simulink model "Vfinal"  (R2023b)
settings: Solver=VariableStepAuto  StartTime=0.0  StopTime=10.0  RelTol=1e-3
settings Model: Creator=meghn  LastModifiedBy=Hp

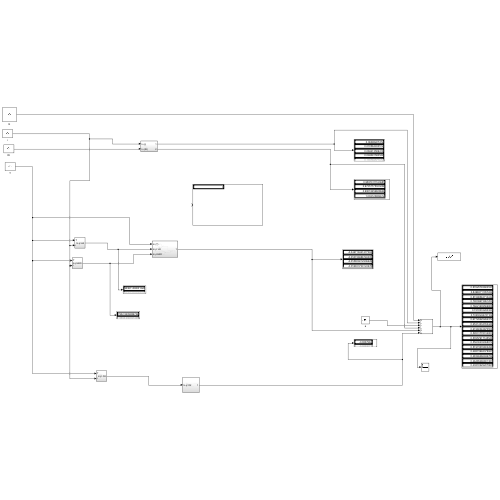
[thumbnail: Simulink's stored preview of the top-level diagram]
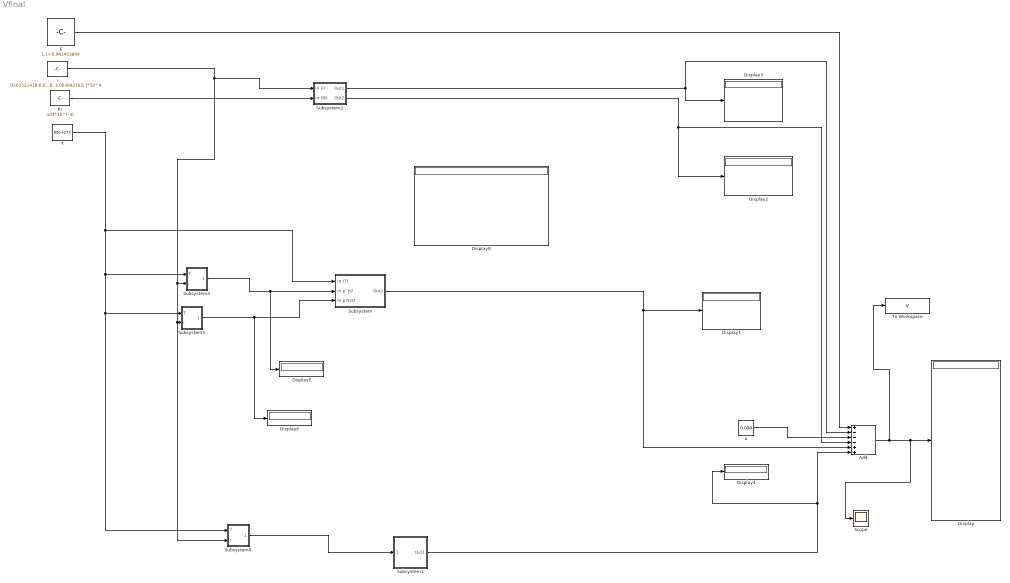
== system Vfinal ==
  Add : Sum  Inputs=+---++
  Display{,1..6,8} (8 alike) : Display
  E : Constant  Value=1.1+0.941453849
  Ri : Constant  Value=.104*10^(-4)
  Scope : Scope
  Subsystem : Subsystem
  Subsystem1 : Subsystem
  Subsystem2 : Subsystem
  Subsystem4 : Subsystem
  Subsystem5 : Subsystem
  Subsystem6 : Subsystem
  T : Constant  Value=800+273
  To Workspace : ToWorkspace  VariableName=V  SampleTime=-1
      settings: Save2DSignal=2-D array (concatenate along first dimension)
  a : Constant  Value=0.094
  i : Constant  Value=|
      | [0.61521418;0.697932053;
      | 0.811669129;
      | 0.904726736;
      | 0.997784343;
      | 1.158050222;
      | 1.26661743;
      | 1.380354505;
      | 1.499261448;
      | 1.659527326;
      | 1.783604136;
      | 1.88183161;
      | 1.990398818;
      | 2.192023634;
      | 2.310930576;
      | 2.398818316;
      | 2.507385524;
      | 2.662481536;
      | 3.003692762;
      | ]*10^4
  wires:
  a/1 -> Add/3
  T/1 -> Subsystem6/1(T), Subsystem5/1(T), Subsystem4/1(T), Subsystem/1(In (T))
  Subsystem4/1(In p' H2) -> Display5/1, Subsystem/2(In p' H2)
  Subsystem5/1(In p'H2O) -> Display6/1, Subsystem/3(In p'H2O)
  Subsystem/1(Out1) -> Display1/1, Add/5
  Subsystem1/1(Out1) -> Display4/1, Add/6
  Subsystem6/1(In p' O2) -> Subsystem1/1(In p' O2)
  Subsystem2/2(Out2) -> Display2/1, Add/4
  Subsystem2/1(Out1) -> Add/2, Display3/1
  i/1 -> Subsystem6/2(i), Subsystem5/2(i), Subsystem4/2(i), Subsystem2/1(In (i))
  Ri/1 -> Subsystem2/2(In (Ri))
  E/1 -> Add/1
  Add/1 -> To Workspace/1, Scope/1, Display/1

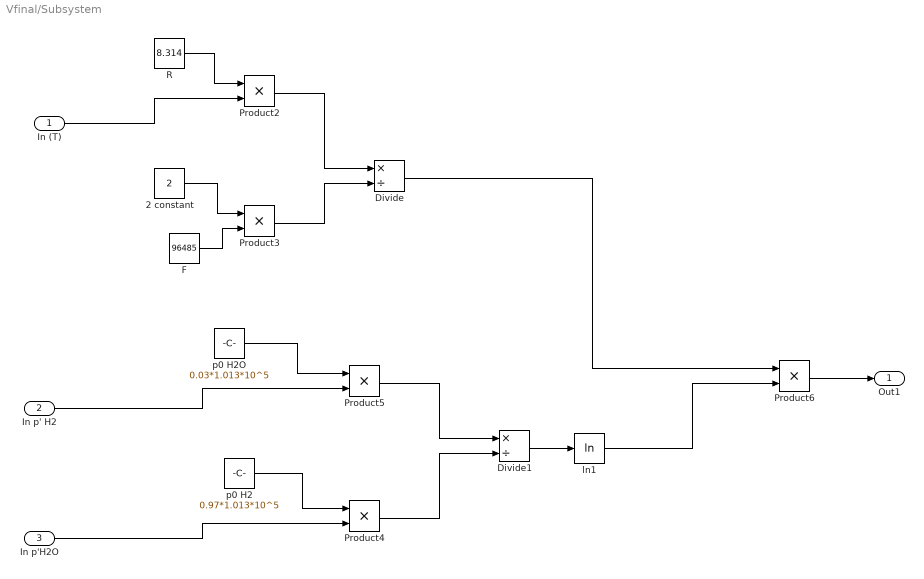
== system Vfinal/Subsystem ==
  In (T) : Inport
  In p' H2 : Inport  Port=2
  In p'H2O : Inport  Port=3
  2 constant : Constant  Value=2
  Divide : Product  Inputs=*/
  Divide1 : Product  Inputs=*/
  F : Constant  Value=96485
  Product{2..6} (5 alike) : Product
  R : Constant  Value=8.314
  ln1 : Math  Operator=log
  p0 H2 : Constant  Value=0.97*1.013*10^5
  p0 H2O : Constant  Value=0.03*1.013*10^5
  Out1 : Outport
  wires:
  Product5/1 -> Divide1/1
  Product4/1 -> Divide1/2
  R/1 -> Product2/1
  ln1/1 -> Product6/2
  In p' H2/1 -> Product5/2
  F/1 -> Product3/2
  Product3/1 -> Divide/2
  p0 H2/1 -> Product4/1
  Divide1/1 -> ln1/1
  p0 H2O/1 -> Product5/1
  Divide/1 -> Product6/1
  2 constant/1 -> Product3/1
  Product2/1 -> Divide/1
  In p'H2O/1 -> Product4/2
  In (T)/1 -> Product2/2
  Product6/1 -> Out1/1

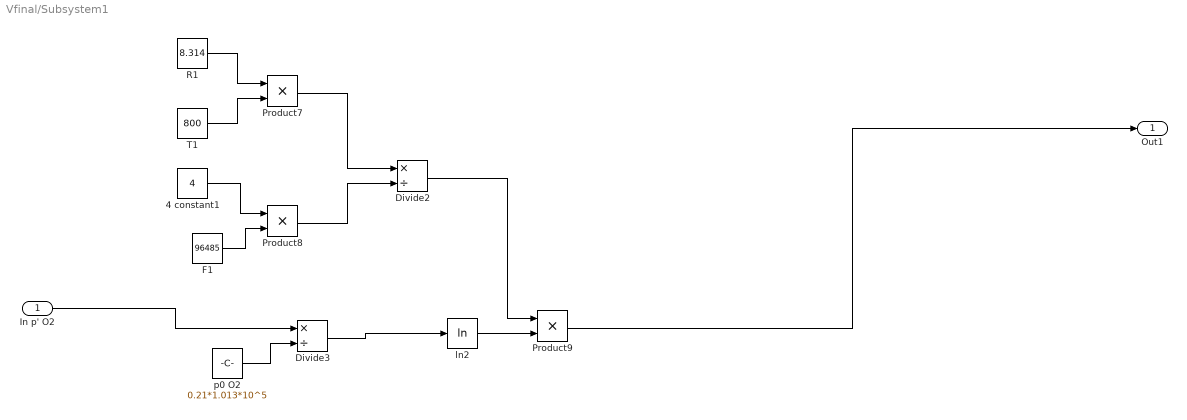
== system Vfinal/Subsystem1 ==
  In p' O2 : Inport
  4 constant1 : Constant  Value=4
  Divide2 : Product  Inputs=*/
  Divide3 : Product  Inputs=*/
  F1 : Constant  Value=96485
  Product7 : Product
  Product8 : Product
  Product9 : Product
  R1 : Constant  Value=8.314
  T1 : Constant  Value=800
  ln2 : Math  Operator=log
  p0 O2 : Constant  Value=0.21*1.013*10^5
  Out1 : Outport
  wires:
  ln2/1 -> Product9/2
  4 constant1/1 -> Product8/1
  R1/1 -> Product7/1
  Divide2/1 -> Product9/1
  p0 O2/1 -> Divide3/2
  F1/1 -> Product8/2
  T1/1 -> Product7/2
  Divide3/1 -> ln2/1
  Product8/1 -> Divide2/2
  Product7/1 -> Divide2/1
  In p' O2/1 -> Divide3/1
  Product9/1 -> Out1/1

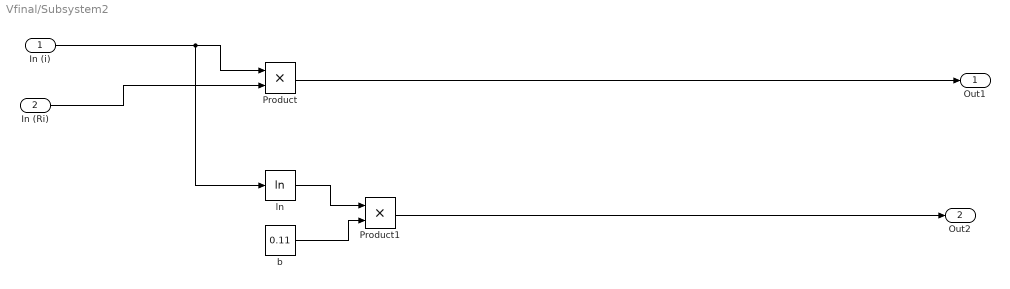
== system Vfinal/Subsystem2 ==
  In (i) : Inport
  In (Ri) : Inport  Port=2
  Product : Product
  Product1 : Product
  b : Constant  Value=0.11
  ln : Math  Operator=log
  Out1 : Outport
  Out2 : Outport  Port=2
  wires:
  b/1 -> Product1/2
  ln/1 -> Product1/1
  Product1/1 -> Out2/1
  In (Ri)/1 -> Product/2
  In (i)/1 -> ln/1, Product/1
  Product/1 -> Out1/1

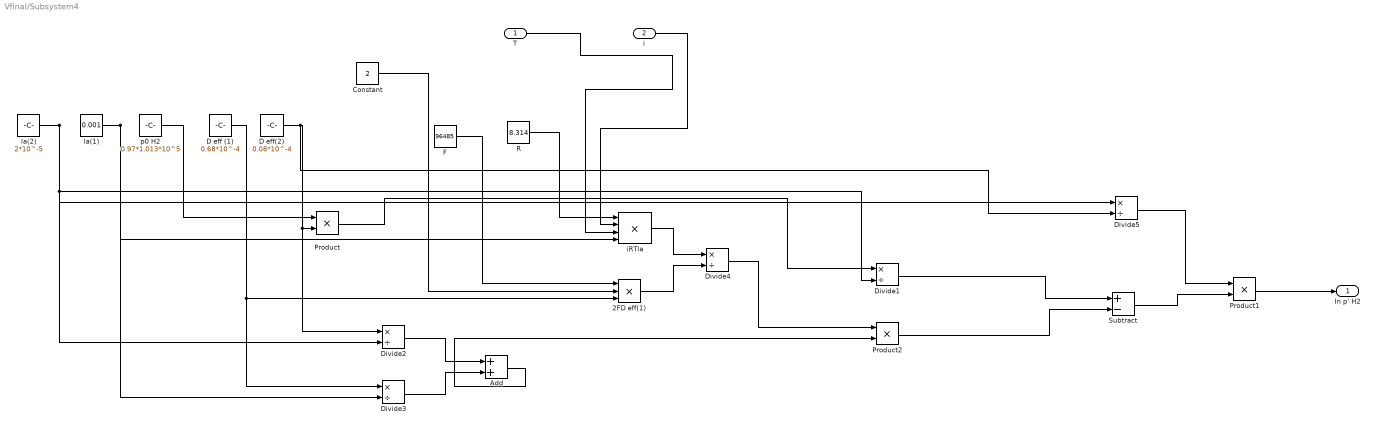
== system Vfinal/Subsystem4 ==
  T : Inport
  i : Inport  Port=2
  2FD eff(1) : Product  Inputs=3  RndMeth=Round
  Add : Sum
  Constant : Constant  Value=2
  D eff (1) : Constant  Value=0.68*10^-4
  D eff(2) : Constant  Value=0.08*10^-4
  Divide{1..5} (5 alike) : Product  Inputs=*/
  F : Constant  Value=96485
  Product : Product
  Product1 : Product
  Product2 : Product
  R : Constant  Value=8.314
  Subtract : Sum  Inputs=+-
  iRTla : Product  Inputs=4
  la(1) : Constant  Value=0.001
  la(2) : Constant  Value=2*10^-5
  p0 H2 : Constant  Value=0.97*1.013*10^5
  In p' H2 : Outport
  wires:
  la(2)/1 -> Divide5/1, Divide2/2, Divide1/2
  D eff(2)/1 -> Divide5/2, Divide2/1, Product/2
  p0 H2/1 -> Product/1
  Product2/1 -> Subtract/2
  Divide3/1 -> Add/2
  F/1 -> 2FD eff(1)/1
  Divide2/1 -> Add/1
  la(1)/1 -> iRTla/4, Divide3/2
  Constant/1 -> 2FD eff(1)/2
  Divide5/1 -> Product1/1
  Divide4/1 -> Product2/1
  Product/1 -> Divide1/1
  R/1 -> iRTla/1
  Add/1 -> Product2/2
  iRTla/1 -> Divide4/1
  i/1 -> iRTla/2
  D eff (1)/1 -> 2FD eff(1)/3, Divide3/1
  Subtract/1 -> Product1/2
  Divide1/1 -> Subtract/1
  T/1 -> iRTla/3
  2FD eff(1)/1 -> Divide4/2
  Product1/1 -> In p' H2/1

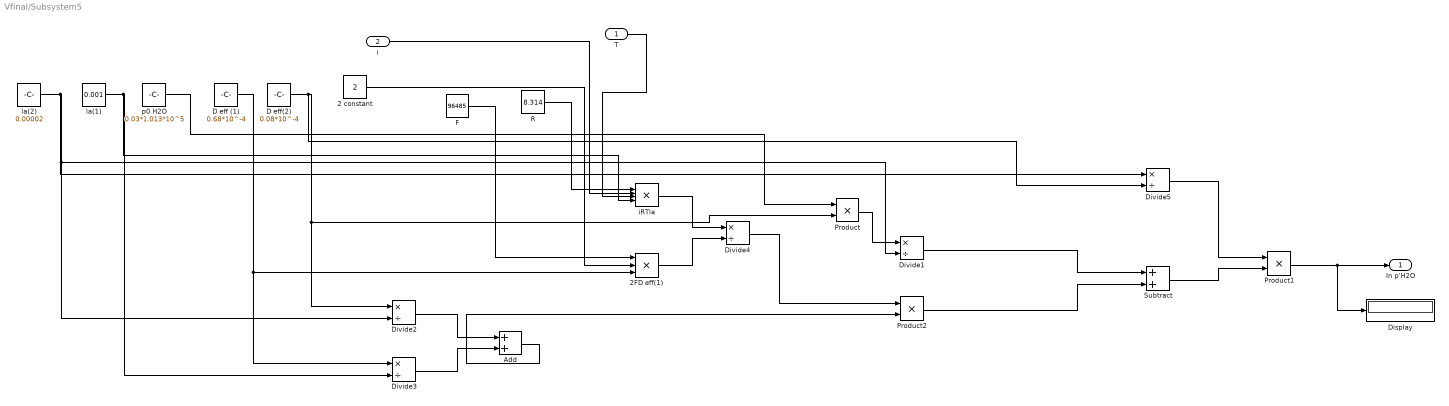
== system Vfinal/Subsystem5 ==
  T : Inport
  i : Inport  Port=2
  2 constant : Constant  Value=2
  2FD eff(1) : Product  Inputs=3  RndMeth=Round
  Add : Sum
  D eff (1) : Constant  Value=0.68*10^-4
  D eff(2) : Constant  Value=0.08*10^-4
  Display : Display
  Divide{1..5} (5 alike) : Product  Inputs=*/
  F : Constant  Value=96485
  Product : Product
  Product1 : Product
  Product2 : Product
  R : Constant  Value=8.314
  Subtract : Sum
  iRTla : Product  Inputs=4
  la(1) : Constant  Value=0.001
  la(2) : Constant  Value=0.00002
  p0 H2O : Constant  Value=0.03*1.013*10^5
  In p'H2O : Outport
  wires:
  la(1)/1 -> iRTla/4, Divide3/2
  Divide4/1 -> Product2/1
  Divide5/1 -> Product1/1
  i/1 -> iRTla/2
  T/1 -> iRTla/3
  2 constant/1 -> 2FD eff(1)/2
  D eff (1)/1 -> 2FD eff(1)/3, Divide3/1
  2FD eff(1)/1 -> Divide4/2
  D eff(2)/1 -> Divide5/2, Divide2/1, Product/2
  Add/1 -> Product2/2
  Product2/1 -> Subtract/2
  p0 H2O/1 -> Product/1
  la(2)/1 -> Divide5/1, Divide2/2, Divide1/2
  F/1 -> 2FD eff(1)/1
  Divide3/1 -> Add/2
  Subtract/1 -> Product1/2
  Product/1 -> Divide1/1
  R/1 -> iRTla/1
  iRTla/1 -> Divide4/1
  Divide2/1 -> Add/1
  Divide1/1 -> Subtract/1
  Product1/1 -> Display/1, In p'H2O/1

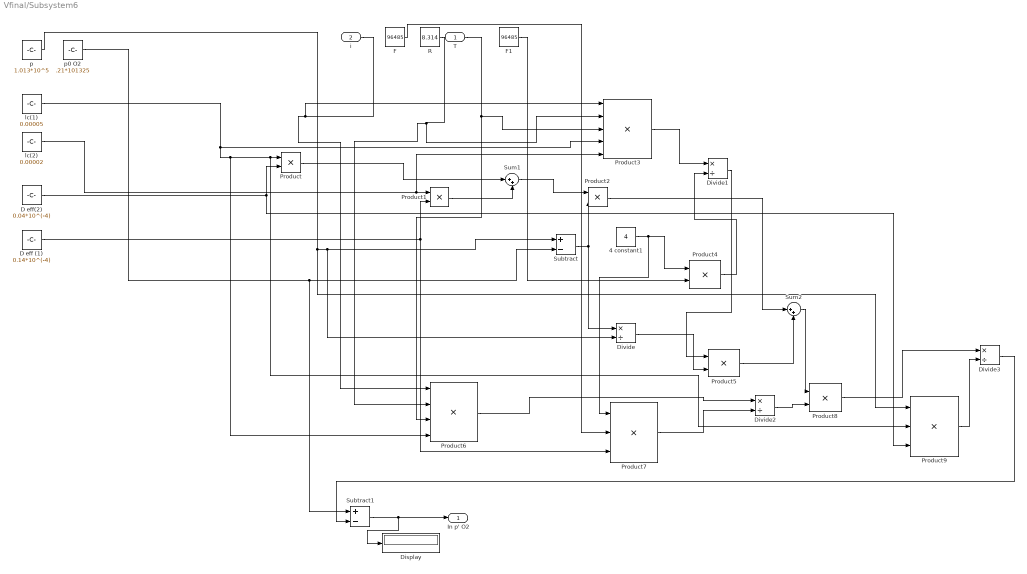
== system Vfinal/Subsystem6 ==
  T : Inport
  i : Inport  Port=2
  4 constant1 : Constant  Value=4
  D eff (1) : Constant  Value=0.14*10^(-4)
  D eff(2) : Constant  Value=0.04*10^(-4)
  Display : Display
  Divide{,1..3} (4 alike) : Product  Inputs=*/
  F : Constant  Value=96485
  F1 : Constant  Value=96485
  Product{,1..2,4..5,8} (6 alike) : Product
  Product3 : Product  Inputs=5
  Product6 : Product  Inputs=4
  Product7 : Product  Inputs=3
  Product9 : Product  Inputs=3
  R : Constant  Value=8.314
  Subtract : Sum  Inputs=+-
  Subtract1 : Sum  Inputs=+-
  Sum1 : Sum  Inputs=|++
  Sum2 : Sum  Inputs=|++
  lc(1) : Constant  Value=0.00005
  lc(2) : Constant  Value=0.00002
  p : Constant  Value=1.013*10^5
  p0 O2 : Constant  Value=.21*101325
  In p' O2 : Outport
  wires:
  lc(1)/1 -> Product6/4, Product9/2, Product/1, Product3/4
  T/1 -> Product6/3, Product3/3
  Subtract1/1 -> Display/1, In p' O2/1
  Product8/1 -> Divide3/1
  Divide1/1 -> Product5/1
  Product6/1 -> Divide2/1
  p/1 -> Product9/1, Divide/2, Subtract/1
  Divide2/1 -> Product8/2
  F1/1 -> Product4/2
  Subtract/1 -> Product2/2, Divide/1
  Product3/1 -> Divide1/1
  R/1 -> Product6/2, Product3/2
  4 constant1/1 -> Product7/1, Product4/1
  lc(2)/1 -> Product3/5, Product1/1
  i/1 -> Product6/1, Product3/1
  D eff (1)/1 -> Product1/2, Product7/3
  Divide3/1 -> Subtract1/2
  D eff(2)/1 -> Product/2, Product9/3
  Product7/1 -> Divide2/2
  Product2/1 -> Sum2/1
  Divide/1 -> Product5/2
  Product5/1 -> Sum2/2
  Product4/1 -> Divide1/2
  Product9/1 -> Divide3/2
  Product1/1 -> Sum1/2
  p0 O2/1 -> Subtract1/1, Subtract/2
  Product/1 -> Sum1/1
  F/1 -> Product7/2
  Sum1/1 -> Product2/1
  Sum2/1 -> Product8/1
